simulink model "ModelloUniciclo"  (R2020a)
settings: Solver=VariableStepAuto  StartTime=0.0  StopTime=10.0  RelTol=1e-3
libraries: mpclib x1
settings Model: Creator=francesco  LastModifiedBy=francesco

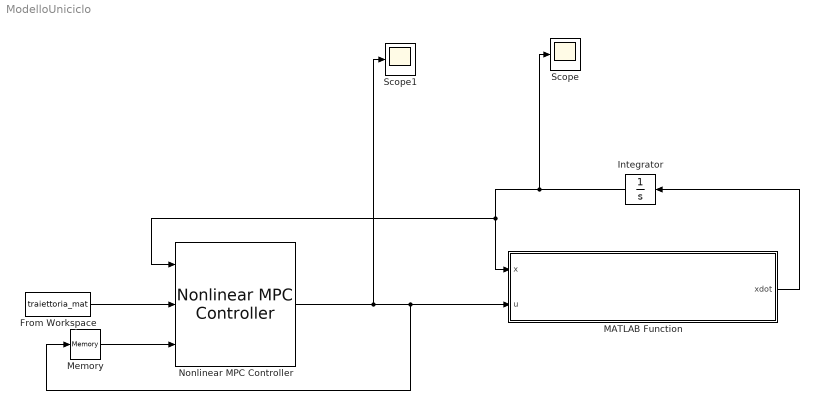
== system ModelloUniciclo ==
  From Workspace : FromWorkspace  VariableName=traiettoria_mat
  Integrator : Integrator
  MATLAB Function : MATLAB Function  TreatAsAtomicUnit=on
  Memory : Memory
  Nonlinear MPC Controller : mpclib/Nonlinear MPC Controller  SCDEnableBlockLinearizationSpecification=on  nlmpcobj=nlobj  UseObjectTs=on  UseMEX=off  md_enabled=off  mvtarget_enabled=off  param_enabled=off  cost_enabled=off  mvseq_enabled=off  stateseq_enabled=off  ovseq_enabled=off  slack_enabled=off  status_enabled=off  ov_min=off  ov_max=off  mv_min=off  mv_max=off  mvrate_min=off  mvrate_max=off  state_min=off  state_max=off  ov_weight=off  mv_weight=off  mvrate_weight=off  ecr_weight=off  nlp_initialize=off
  Scope : Scope
  Scope1 : Scope
  wires:
  Nonlinear MPC Controller/1 -> Scope1/1, Memory/1, MATLAB Function/2(u)
  MATLAB Function/1(xdot) -> Integrator/1
  Integrator/1 -> Scope/1, MATLAB Function/1(x), Nonlinear MPC Controller/1
  Memory/1 -> Nonlinear MPC Controller/3
  From Workspace/1 -> Nonlinear MPC Controller/2

== matlab function ModelloUniciclo/MATLAB Function ==
  data: x input; u input; xdot output
function xdot  = ModelloCinematicoVeicolo(x,u)

    %L=params.Vehicle_Length;
%     x_update = [cos(x(3))*x(4);
%                 sin(x(3))*x(4);
%                 (tan(u(2))/L)*x(4);
%                 0.5*u(1)];

%     x_update = [u(1) * cos(x(3)) * cos(u(2));
%                 u(1) * sin(x(3)) * cos(u(2));
%                 u(1)/L * sin(u(2))
%                 0.5*u(1)];

     L=4;
     xdot=[u(1)*cos(x(3));
         u(1)*sin(x(3));
         (atan2(x(4))/L)*u(1);
         u(2)];
%      stato=x,y,teta,psi ingressi=v,w


    
    
    
    
end
